simulink model "P1simulink2022a"  (R2022a)
settings: Solver=VariableStepAuto  StartTime=0.0  StopTime=20  RelTol=1e-3
values from neighbouring files (symbols this model uses):
  K = -0.8    [P1.m]    (also in P2.m = -1; P4.m; TestGraph.m; ZenoPlot.m)
  V = 0    [P1.m]    (also in P2.m = 15; P3.m = 15; P4.m = 15; QuiverTest.m = zeros(length(U),length(U)) -g)
libraries: simulink x1
settings Model: Creator=TERESA NOGUEIRA  LastModifiedBy=João
settings ModelReferenceCC: EnableRefExpFcnMdlSchedulingChecks=off
settings RTWCC: Description=Generic Real-Time Target

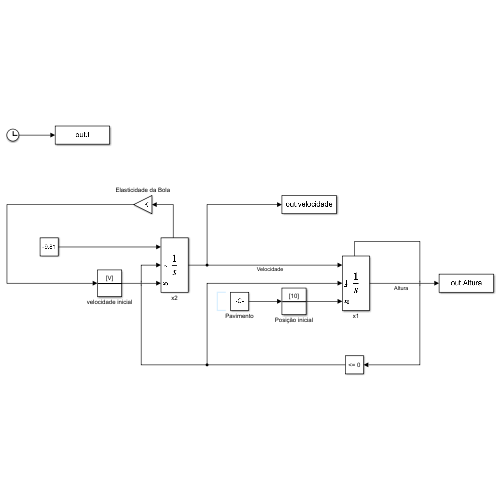
[thumbnail: Simulink's stored preview of the top-level diagram]
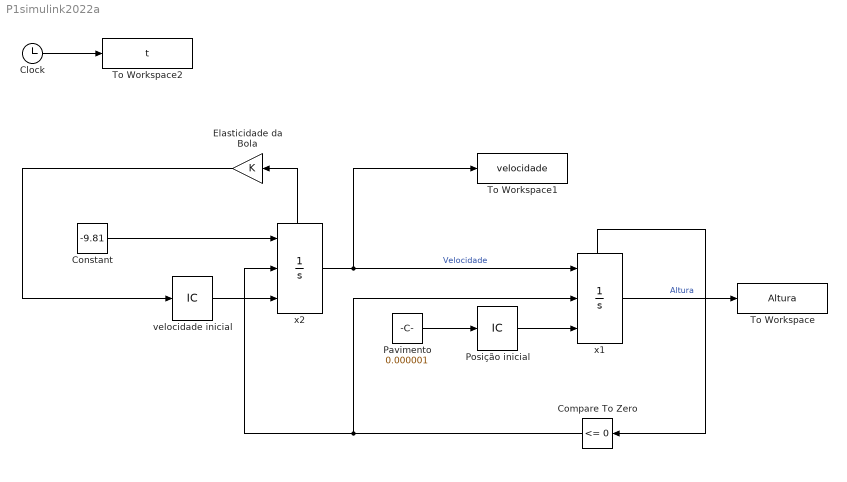
== system P1simulink2022a ==
  Clock : Clock
      settings: Decimation=200
  Compare To Zero : simulink/Logic and Bit Operations/Compare To Zero  relop=<=  OutDataTypeStr=boolean
  Constant : Constant  Value=-9.81
  Elasticidade da Bola : Gain  Gain=K
  Pavimento : Constant  Value=0.000001
  Posição inicial : InitialCondition  Value=10
  To Workspace : ToWorkspace  VariableName=Altura  SampleTime=-1
      settings: Save2DSignal=2-D array (concatenate along first dimension)
  To Workspace1 : ToWorkspace  VariableName=velocidade  SampleTime=-1
      settings: Save2DSignal=2-D array (concatenate along first dimension)
  To Workspace2 : ToWorkspace  VariableName=t  SampleTime=-1
      settings: Save2DSignal=2-D array (concatenate along first dimension)
  velocidade inicial : InitialCondition  Value=V
  x1 : Integrator  ExternalReset=rising  InitialConditionSource=external  ShowStatePort=on
  x2 : Integrator  ExternalReset=rising  InitialConditionSource=external  ShowStatePort=on
  wires:
  x1/State -> Compare To Zero/1
  Compare To Zero/1 -> x2/2, x1/2
  x1/1 -> To Workspace/1  "Altura"
  Pavimento/1 -> Posição inicial/1
  Clock/1 -> To Workspace2/1
  x2/State -> Elasticidade da Bola/1
  Elasticidade da Bola/1 -> velocidade inicial/1
  Constant/1 -> x2/1
  Posição inicial/1 -> x1/3
  x2/1 -> To Workspace1/1, x1/1  "Velocidade"
  velocidade inicial/1 -> x2/3
